simulink model "Full_System_REF"  (R2025b)
settings: Solver=VariableStepAuto  StartTime=0.0  StopTime=tspan  RelTol=rel_tol  AbsTol=abs_tol
settings Model: Creator=koryh  LastModifiedBy=kjhaydon

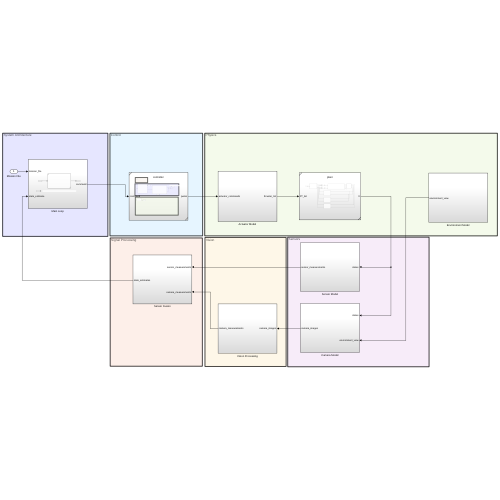
[thumbnail: Simulink's stored preview of the top-level diagram]
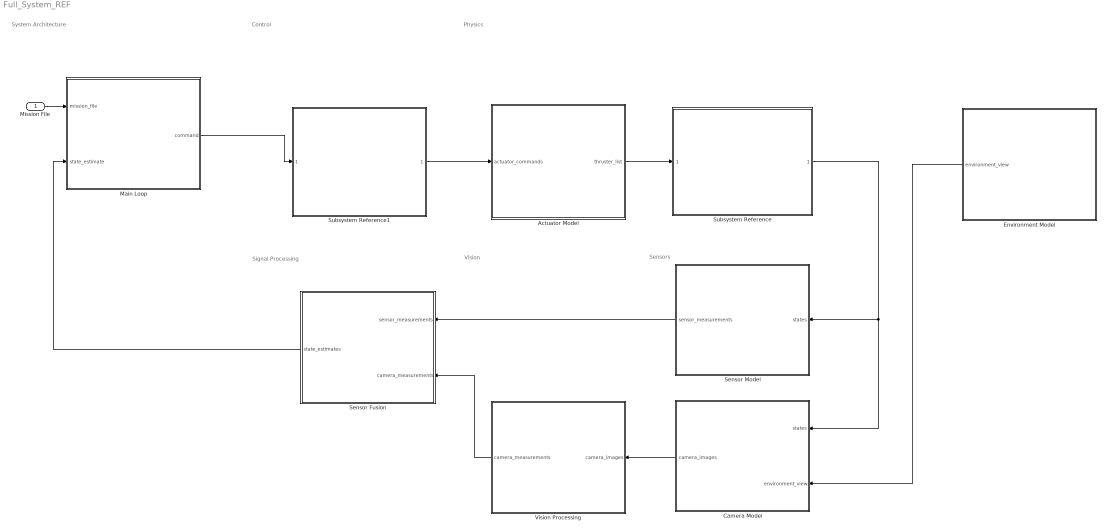
== system Full_System_REF ==
  note: Signal Processing
  note: Vision
  note: Sensors
  note: Physics
  note: Control
  note: System Architecture
  Mission File : Inport
  Actuator Model : Subsystem
  Camera Model : Subsystem
  Environment Model : Subsystem
  Main Loop : Subsystem
  Sensor Fusion : Subsystem
  Sensor Model : Subsystem
  Subsystem Reference : Subsystem  ReferencedSubsystem=plant
  Subsystem Reference1 : Subsystem  ReferencedSubsystem=controller
  Vision Processing : Subsystem
  wires:
  Mission File/1 -> Main Loop/1(mission_file)
  Subsystem Reference1/1 -> Actuator Model/1(actuator_commands)
  Environment Model/1(environment_view) -> Camera Model/2(environment_view)
  Camera Model/1(camera_images) -> Vision Processing/1(camera_images)
  Sensor Model/1(sensor_measurements) -> Sensor Fusion/1(sensor_measurements)
  Vision Processing/1(camera_measurements) -> Sensor Fusion/2(camera_measurements)
  Sensor Fusion/1(state_estimates) -> Main Loop/2(state_estimate)
  Main Loop/1(command) -> Subsystem Reference1/1
  Actuator Model/1(thruster_list) -> Subsystem Reference/1
  Subsystem Reference/1 -> Camera Model/1(states), Sensor Model/1(states)

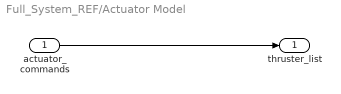
== system Full_System_REF/Actuator Model ==
  actuator_commands : Inport
  thruster_list : Outport
  wires:
  actuator_commands/1 -> thruster_list/1

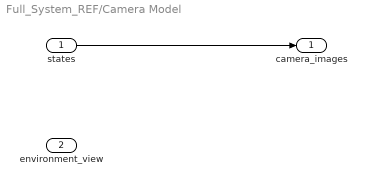
== system Full_System_REF/Camera Model ==
  states : Inport
  environment_view : Inport  Port=2
  camera_images : Outport
  wires:
  states/1 -> camera_images/1

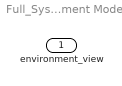
== system Full_System_REF/Environment Model ==
  environment_view : Outport

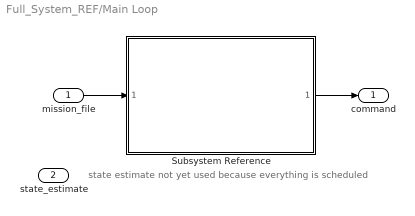
== system Full_System_REF/Main Loop ==
  note: state estimate not yet used because everything is scheduled
  mission_file : Inport
  state_estimate : Inport  Port=2
  Subsystem Reference : Subsystem  ReferencedSubsystem=mission_file_parser
  command : Outport
  wires:
  mission_file/1 -> Subsystem Reference/1
  Subsystem Reference/1 -> command/1

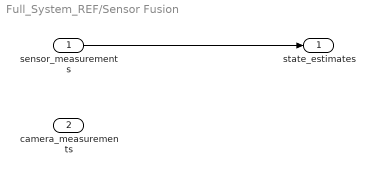
== system Full_System_REF/Sensor Fusion ==
  sensor_measurements : Inport
  camera_measurements : Inport  Port=2
  state_estimates : Outport
  wires:
  sensor_measurements/1 -> state_estimates/1

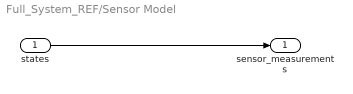
== system Full_System_REF/Sensor Model ==
  states : Inport
  sensor_measurements : Outport
  wires:
  states/1 -> sensor_measurements/1

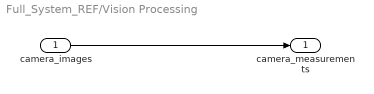
== system Full_System_REF/Vision Processing ==
  camera_images : Inport
  camera_measurements : Outport
  wires:
  camera_images/1 -> camera_measurements/1
